simulink model "simulink"  (R2025b)
settings: Solver=ode4  StartTime=0.0  StopTime=2  FixedStep=1e-3  RelTol=1e-3
values from neighbouring files (symbols this model uses):
  k = db2mag(18)    [controlador.m]    (also in diseno_observador.m = 0.0083317)
libraries: cstblocks x2
settings Model: Creator=rocio  LastModifiedBy=bianc
settings DebuggingCC: UnconnectedInputMsg=warning  UnconnectedOutputMsg=warning  UnconnectedLineMsg=warning
settings ModelReferenceCC: EnableRefExpFcnMdlSchedulingChecks=on
settings RTWCC: GPUComputeCapability=3.5  DLArmComputeVersion=19.05

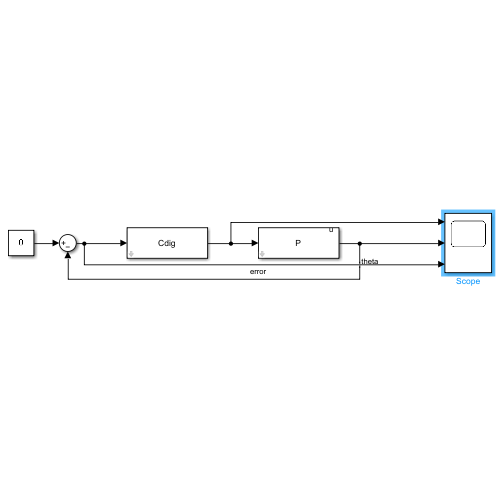
[thumbnail: Simulink's stored preview of the top-level diagram]
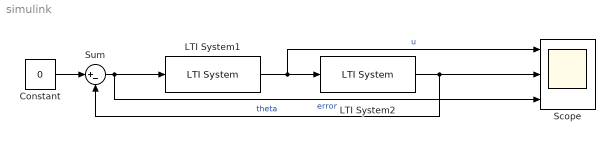
== system simulink ==
  Constant : Constant  Value=0
  LTI System1 : cstblocks/LTI System  sys=Cdig  IC=[]  PadeOrder=0
  LTI System2 : cstblocks/LTI System  sys=P  IC=[(6*pi/180)/k 0]  PadeOrder=0
  Scope : Scope  NumInputPorts=3
      settings: ActiveDisplayYMinimum=-3.9352913155162721  ActiveDisplayYMaximum=20.233942519567265
  Sum : Sum  Inputs=|+-
  wires:
  Constant/1 -> Sum/1
  Sum/1 -> LTI System1/1, Scope/3  "error"
  LTI System2/1 -> Sum/2, Scope/2  "theta"
  LTI System1/1 -> Scope/1, LTI System2/1  "u"
